simulink model "New_density"  (R2013b)
settings: Solver=FixedStepDiscrete  StartTime=0.0  StopTime=0  FixedStep=1  RelTol=1e-3
libraries: carnot x1
settings Model: DEBUGGLOBALLEVEL=1  DEBUGWRITETOFILE=0  DEBUGFILENAME=bla.txt  DEBUGMAXCONSECUTIVEWARNINGS=inf  DEBUGMAXTOTALWARNINGS=inf  Creator=awohlfei  LastModifiedBy=awohlfei
settings OptimizationCC: ExpressionDepthLimit=2147483647
settings DebuggingCC: UnderspecifiedInitializationDetection=Simplified  MergeDetectMultiDrivingBlocksExec=error  StateNameClashWarn=warning

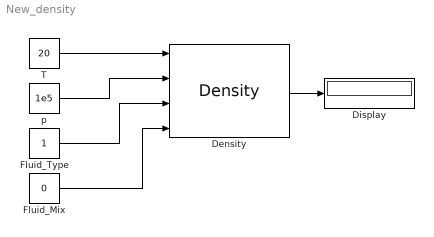
== system New_density ==
  Density : carnot/Basic/Material_Properties/Density  VariantControl=CarlibClassic  INPUTARGUMENTS=state variables (classic)  DEBUGLEVEL=DEBUGLEVEL  MAXTOTALWARNINGS=inf  MAXCONSECUTIVEWARNINGS=inf  WRITETOFILE=0  FILENAME='errors.txt'
  Display : Display
  Fluid_Mix : Constant  Value=0
  Fluid_Type : Constant
  T : Constant  Value=20
  p : Constant  Value=1e5
  wires:
  T/1 -> Density/1
  p/1 -> Density/2
  Fluid_Type/1 -> Density/3
  Fluid_Mix/1 -> Density/4
  Density/1 -> Display/1
